simulink model "Adaptive_Simulation"  (R2018a)
settings: Solver=VariableStepAuto  StartTime=0.0  StopTime=100  RelTol=1e-3
values from neighbouring files (symbols this model uses):
  Am = [0 1; -(nat_freq^2) -2*damping_rat*nat_freq]    [AdaptiveFullState.m]    (also in Test1.m = [0 1; -(wm^2) -2*c*wm]; ThetaPlot.m)
  aug_theta_star = [Theta_x_star;Theta_r_star]    [AdaptiveFullState.m]
  B = [0;1]    [AdaptiveFullState.m]    (also in ThetaPlot.m)
  Gamma = [3 0 0;0 0.5 0;0 0 2]    [AdaptiveFullState.m]    (also in LyapunovCheck.m = eye(3))
  gm = nat_freq^2    (= 4)    [AdaptiveFullState.m]    (also in Test1.m = [0;wm^2]; ThetaPlot.m)
  Kp = Kpvec(1)    [AdaptiveFullState.m]    (also in ThetaPlot.m)
  Ktheta = Fittheta(1)    [AdaptiveFullState.m]    (also in Test1.m = polyfit(xrad,x1,1))
  Kw = Fitw(1)    [AdaptiveFullState.m]
  P = lyap(Am',Q)    [AdaptiveFullState.m]    (also in LyapunovCheck.m = eye(2); Test1.m)
  tau = 0.31    [AdaptiveFullState.m]    (also in Test1.m; ThetaPlot.m)
libraries: simulink x2, simulink_extras x1
settings Model: Creator=ageng  LastModifiedBy=ageng
settings SolverCC: ZeroCrossAlgorithm=Adaptive
settings DebuggingCC: AlgebraicLoopMsg=none

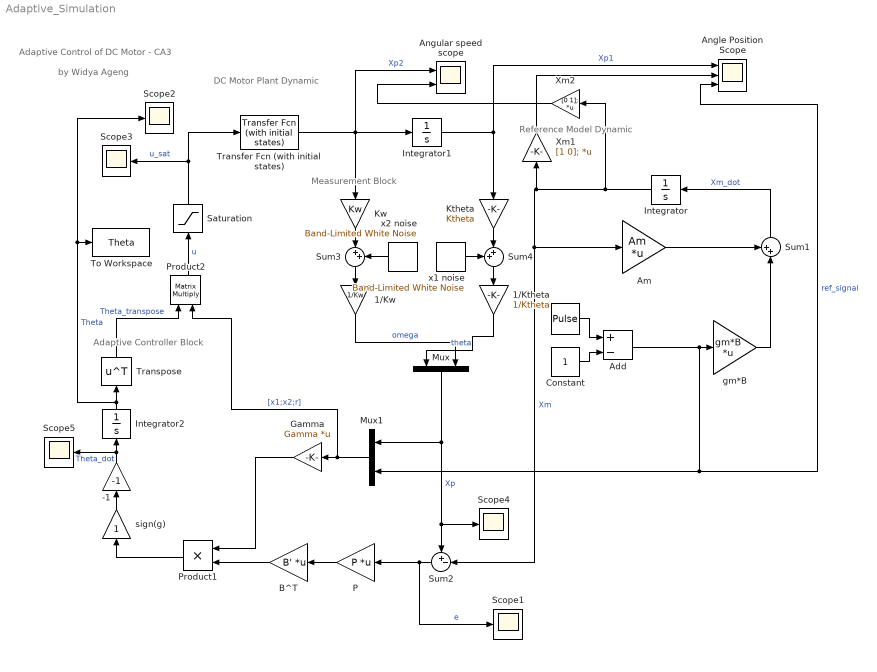
== system Adaptive_Simulation ==
  note: DC Motor Plant Dynamic
  note: Measurement Block
  note: Adaptive Controller Block
  note: Reference Model Dynamic
  note: by Widya Ageng
  note: Adaptive Control of DC Motor - CA3
  " " : DiscretePulseGenerator  PulseType=Time based  Amplitude=2  Period=10  PulseWidth=50
  "-1 " : Gain  Gain=-1
  1/Ktheta : Gain  Gain=1/Ktheta
  1/Kw : Gain  Gain=1/Kw
  Add : Sum  Inputs=+-
  Am : Gain  Gain=Am  Multiplication=Matrix(K*u)
  Angle Position Scope : Scope  NumInputPorts=3
  Angular speed scope : Scope  NumInputPorts=2
  B^T : Gain  Gain=B'  Multiplication=Matrix(K*u) (u vector)
  Constant : Constant  SampleTime=Inf
  Gamma : Gain  Gain=Gamma  Multiplication=Matrix(K*u) (u vector)
  Integrator : Integrator  InitialCondition=[0.01;0.01]
  Integrator1 : Integrator
  Integrator2 : Integrator  InitialCondition=aug_theta_star*0
  Ktheta : Gain  Gain=Ktheta
  Kw : Gain  Gain=Kw
  Mux : Mux  Inputs=2
  Mux1 : Mux  Inputs=2
  P : Gain  Gain=P  Multiplication=Matrix(K*u) (u vector)
  Product1 : Product
  Product2 : Product  Multiplication=Matrix(*)
  Saturation : Saturate  UpperLimit=5  LowerLimit=-5
  Scope{1..5} (5 alike) : Scope
  Sum1 : Sum  Inputs=++|
  Sum2 : Sum  Inputs=+-|
  Sum3 : Sum  Inputs=|++
  Sum4 : Sum  Inputs=++|
  To Workspace : ToWorkspace  VariableName=Theta  SaveFormat=Timeseries  SampleTime=-1
      settings: Decimation=3
  Transfer Fcn (with initial states) : simulink_extras/Additional Linear/Transfer Fcn (with initial states)  N=[Kp]  D=[tau 1]  X0=0
  Transpose : Math  Operator=transpose  SaturateOnIntegerOverflow=on
  Xm1 : Gain  Gain=[1 0];  Multiplication=Matrix(K*u) (u vector)
  Xm2 : Gain  Gain=[0 1];  Multiplication=Matrix(K*u) (u vector)
  gm*B : Gain  Gain=gm*B  Multiplication=Matrix(K*u)
  sign(g) : Gain
  x1 noise : simulink/Sources/Band-Limited White Noise  Cov=[1e-6]  Ts=8e-5  seed=[1]
  x2 noise : simulink/Sources/Band-Limited White Noise  Cov=[1e-6]  Ts=8e-5  seed=[1]
  wires:
  Transfer Fcn (with initial states)/1 -> Kw/1, Angular speed scope/1, Integrator1/1  "Xp2"
  Integrator1/1 -> Ktheta/1, Angle Position Scope/1  "Xp1"
  1/Kw/1 -> Mux/2  "omega"
  1/Ktheta/1 -> Mux/1  "theta"
  Mux/1 -> Mux1/1, Scope4/1, Sum2/1  "Xp"
  Add/1 -> Mux1/2, Angle Position Scope/3, gm*B/1  "ref_signal"
  Am/1 -> Sum1/1
  gm*B/1 -> Sum1/2
  Sum1/1 -> Integrator/1  "Xm_dot"
  Integrator/1 -> Xm2/1, Xm1/1, Sum2/2, Am/1  "Xm"
  Sum2/1 -> Scope1/1, P/1  "e"
  P/1 -> B^T/1
  Product1/1 -> sign(g)/1
  sign(g)/1 -> "-1 "/1
  Gamma/1 -> Product1/1
  B^T/1 -> Product1/2
  Mux1/1 -> Product2/2, Gamma/1  "[x1;x2;r]"
  "-1 "/1 -> Integrator2/1, Scope5/1  "Theta_dot"
  Integrator2/1 -> To Workspace/1, Scope2/1, Transpose/1  "Theta"
  Transpose/1 -> Product2/1  "Theta_transpose"
  " "/1 -> Add/1
  Constant/1 -> Add/2
  Xm1/1 -> Angle Position Scope/2
  Product2/1 -> Saturation/1  "u"
  Saturation/1 -> Scope3/1, Transfer Fcn (with initial states)/1  "u_sat"
  x1 noise/1 -> Sum4/1
  x2 noise/1 -> Sum3/2
  Xm2/1 -> Angular speed scope/2
  Ktheta/1 -> Sum4/2
  Sum4/1 -> 1/Ktheta/1
  Kw/1 -> Sum3/1
  Sum3/1 -> 1/Kw/1
